simulink library "Lib_PF_BusSlackAC_TMATS"  (R2017a)
settings: Solver=ode45  StartTime=0.0  StopTime=10.0  RelTol=1e-3  EnableMultiTasking=on
Description:
  | Thomas Modules
settings Model: Creator=jwchapm2  LastModifiedBy=glthoma1
settings DataIOCC: LimitDataPoints=on  SaveFormat=Array
settings OptimizationCC: ExpressionDepthLimit=2147483647  LifeSpan=inf
settings DebuggingCC: UnderspecifiedInitializationDetection=Classic  MergeDetectMultiDrivingBlocksExec=none  SolverPrmCheckMsg=warning  StateNameClashWarn=warning  SFUnexpectedBacktrackingDiag=warning  SFNoUnconditionalDefaultTransitionDiag=warning  SFExecutionAtInitializationDiag=none
settings HardwareCC: ProdBitPerPointer=32  ProdBitPerSizeT=32  ProdBitPerPtrDiffT=32  ProdLargestAtomicFloat=None  ProdIntDivRoundTo=Undefined  ProdEndianess=Unspecified  ProdWordSize=32  ProdHWDeviceType=32-bit Generic
settings ModelReferenceCC: PropagateSignalLabelsOutOfModel=off
settings GRTTargetCC: TargetLangStandard=C89/C90 (ANSI)  GeneratePreprocessorConditionals=Disable all
settings ConfigComp: CovMetricSettings=dw  CovHtmlReporting=on  CovSaveCumulativeToWorkspaceVar=on  CovSaveSingleToWorkspaceVar=on  CovExternalEMLEnable=off

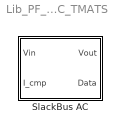
== system Lib_PF_BusSlackAC_TMATS ==
  SlackBus AC : Subsystem

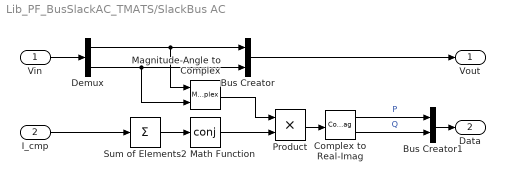
== system Lib_PF_BusSlackAC_TMATS/SlackBus AC ==
  Vin : Inport
  I_cmp : Inport  Port=2
  Bus Creator : BusCreator  Inputs=2
  Bus Creator1 : BusCreator  Inputs=2
  Complex to Real-Imag : ComplexToRealImag
  Demux : Demux  Outputs=2
  Magnitude-Angle to Complex : MagnitudeAngleToComplex
  Math Function : Math  Operator=conj  SaturateOnIntegerOverflow=on
  Product : Product
  Sum of Elements2 : Sum  Inputs=+
  Vout : Outport
  Data : Outport  Port=2
  wires:
  Complex to Real-Imag/2 -> Bus Creator1/2  "Q"
  Complex to Real-Imag/1 -> Bus Creator1/1  "P"
  Product/1 -> Complex to Real-Imag/1
  Math Function/1 -> Product/2
  Magnitude-Angle to Complex/1 -> Product/1
  Sum of Elements2/1 -> Math Function/1
  I_cmp/1 -> Sum of Elements2/1
  Demux/2 -> Bus Creator/2, Magnitude-Angle to Complex/2
  Demux/1 -> Bus Creator/1, Magnitude-Angle to Complex/1
  Bus Creator/1 -> Vout/1
  Bus Creator1/1 -> Data/1
  Vin/1 -> Demux/1
